simulink model "Plant_s"  (R2023a)
settings: Solver=VariableStepAuto  StartTime=0.0  StopTime=10.0  RelTol=1e-3
undefined symbols (not defined in the file): c, C, C_alpha_f, C_col, C_r, E, e_p0, F_zf, F_zr, Iz, J_col, K, l_f, l_r, m, n_st, T_f
settings Model: Creator=Tan_Tram  LastModifiedBy=Tan_Tram

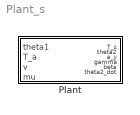
== system Plant_s ==
  Plant : Subsystem

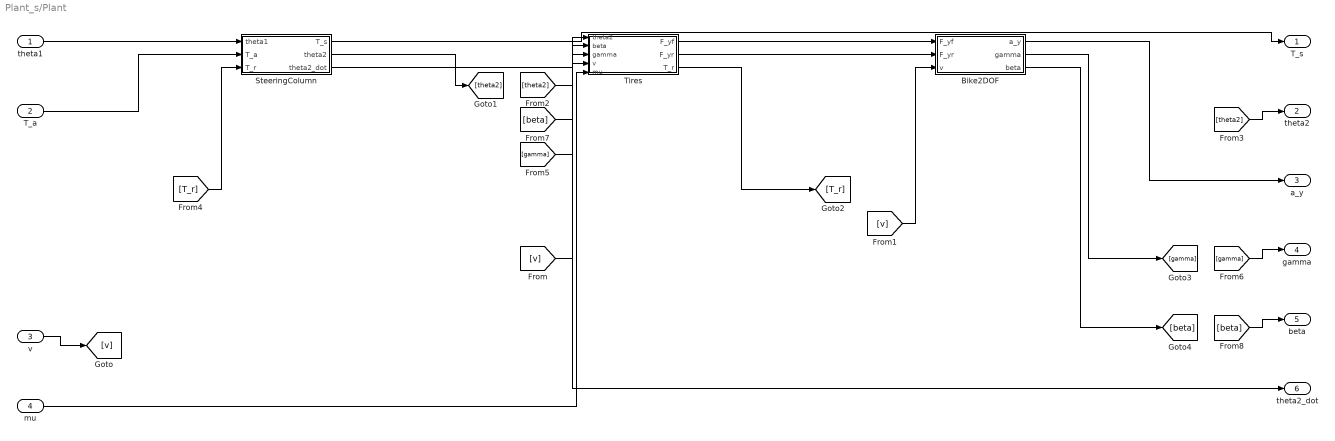
== system Plant_s/Plant ==
  theta1 : Inport
  T_a : Inport  Port=2
  v : Inport  Port=3
  mu : Inport  Port=4
  Bike2DOF : Subsystem
  SteeringColumn : Subsystem
  Tires : Subsystem
  T_s : Outport
  theta2 : Outport  Port=2
  a_y : Outport  Port=3
  gamma : Outport  Port=4
  beta : Outport  Port=5
  theta2_dot : Outport  Port=6
  wires:
  theta1/1 -> SteeringColumn/1(theta1)
  T_a/1 -> SteeringColumn/2(T_a)
  mu/1 -> Tires/5(mu)
  Tires/1(F_yf) -> Bike2DOF/1(F_yf)
  Tires/2(F_yr) -> Bike2DOF/2(F_yr)
  SteeringColumn/1(T_s) -> T_s/1
  Bike2DOF/1(a_y) -> a_y/1
  SteeringColumn/3(theta2_dot) -> theta2_dot/1
  v/1 -> [v]
  [v] -> Tires/4(v)
  [v] -> Bike2DOF/3(v)
  SteeringColumn/2(theta2) -> [theta2]
  [theta2] -> Tires/1(theta2)
  [theta2] -> theta2/1
  Tires/3(T_r) -> [T_r]
  [T_r] -> SteeringColumn/3(T_r)
  Bike2DOF/2(gamma) -> [gamma]
  [gamma] -> Tires/3(gamma)
  [gamma] -> gamma/1
  Bike2DOF/3(beta) -> [beta]
  [beta] -> Tires/2(beta)
  [beta] -> beta/1

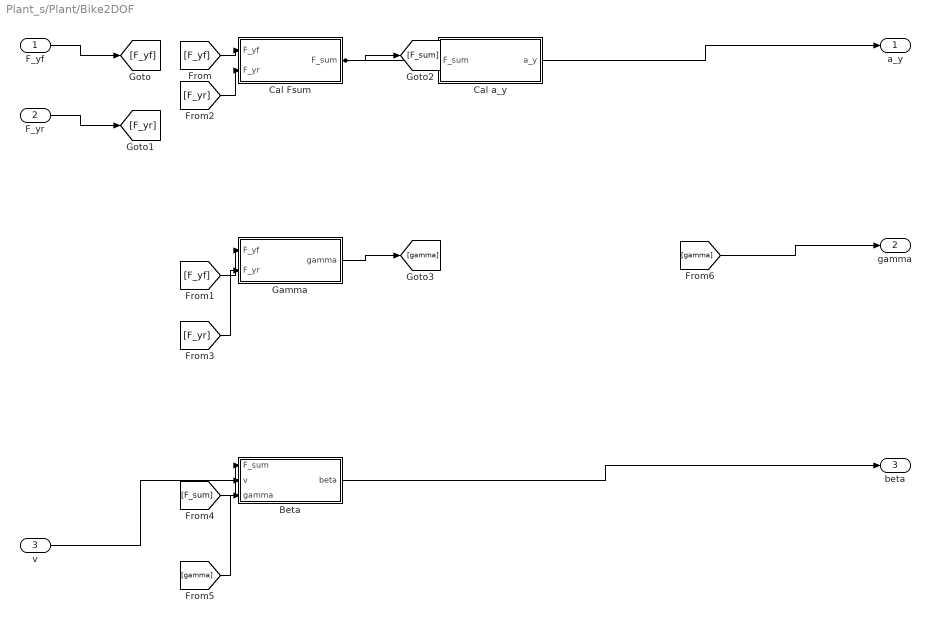
== system Plant_s/Plant/Bike2DOF ==
  F_yf : Inport
  F_yr : Inport  Port=2
  v : Inport  Port=3
  Beta : Subsystem
  Cal Fsum : Subsystem
  Cal a_y : Subsystem
  Gamma : Subsystem
  a_y : Outport
  gamma : Outport  Port=2
  beta : Outport  Port=3
  wires:
  Beta/1(beta) -> beta/1
  v/1 -> Beta/2(v)
  [gamma] -> gamma/1
  [gamma] -> Beta/3(gamma)
  Gamma/1(gamma) -> [gamma]
  Cal a_y/1(a_y) -> a_y/1
  [F_sum] -> Beta/1(F_sum)
  Cal Fsum/1(F_sum) -> [F_sum], Cal a_y/1(F_sum)
  [F_yr] -> Gamma/2(F_yr)
  [F_yr] -> Cal Fsum/2(F_yr)
  F_yr/1 -> [F_yr]
  [F_yf] -> Gamma/1(F_yf)
  [F_yf] -> Cal Fsum/1(F_yf)
  F_yf/1 -> [F_yf]

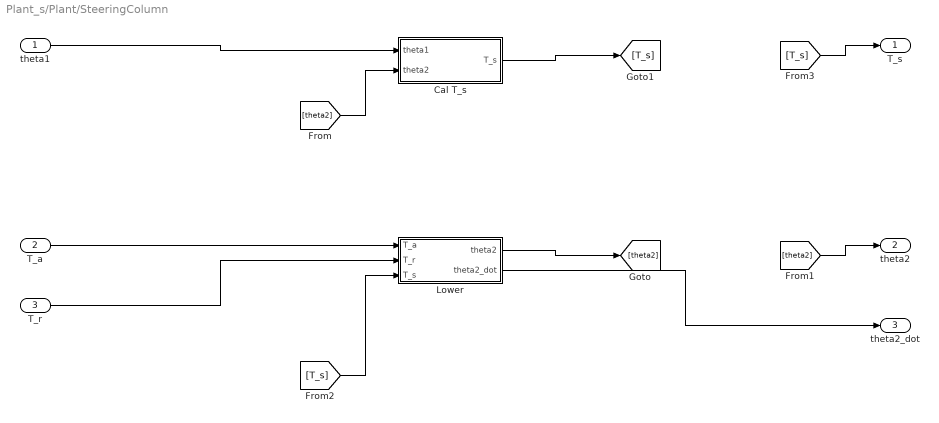
== system Plant_s/Plant/SteeringColumn ==
  theta1 : Inport
  T_a : Inport  Port=2
  T_r : Inport  Port=3
  Cal T_s : Subsystem
  Lower : Subsystem
  T_s : Outport
  theta2 : Outport  Port=2
  theta2_dot : Outport  Port=3
  wires:
  [T_s] -> T_s/1
  [T_s] -> Lower/3(T_s)
  Cal T_s/1(T_s) -> [T_s]
  [theta2] -> theta2/1
  [theta2] -> Cal T_s/2(theta2)
  Lower/1(theta2) -> [theta2]
  Lower/2(theta2_dot) -> theta2_dot/1
  T_r/1 -> Lower/2(T_r)
  T_a/1 -> Lower/1(T_a)
  theta1/1 -> Cal T_s/1(theta1)

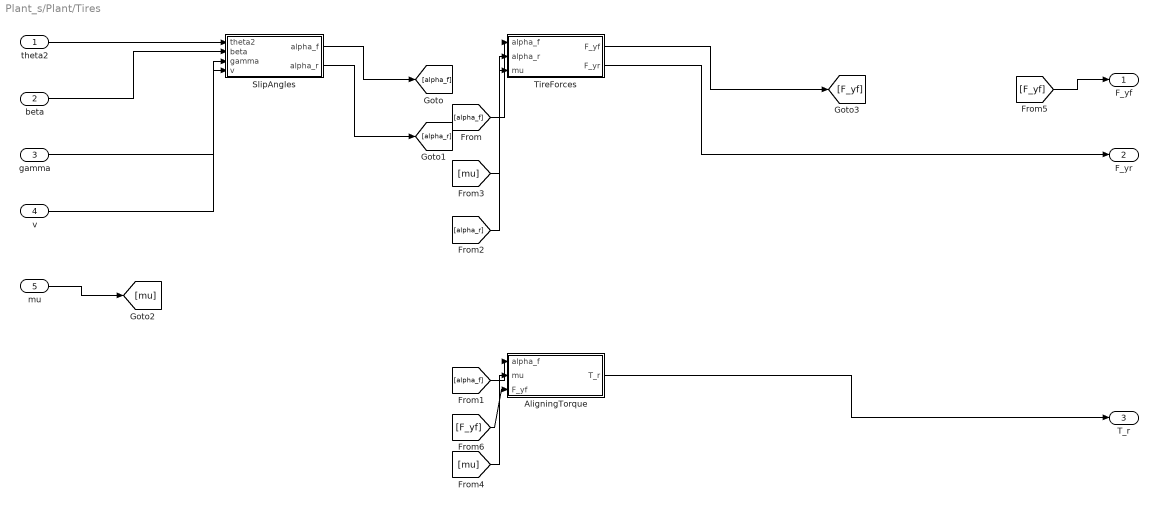
== system Plant_s/Plant/Tires ==
  theta2 : Inport
  beta : Inport  Port=2
  gamma : Inport  Port=3
  v : Inport  Port=4
  mu : Inport  Port=5
  AligningTorque : Subsystem
  SlipAngles : Subsystem
  TireForces : Subsystem
  F_yf : Outport
  F_yr : Outport  Port=2
  T_r : Outport  Port=3
  wires:
  AligningTorque/1(T_r) -> T_r/1
  TireForces/2(F_yr) -> F_yr/1
  [F_yf] -> AligningTorque/3(F_yf)
  [F_yf] -> F_yf/1
  TireForces/1(F_yf) -> [F_yf]
  [mu] -> AligningTorque/2(mu)
  [mu] -> TireForces/3(mu)
  mu/1 -> [mu]
  [alpha_r] -> TireForces/2(alpha_r)
  SlipAngles/2(alpha_r) -> [alpha_r]
  [alpha_f] -> AligningTorque/1(alpha_f)
  [alpha_f] -> TireForces/1(alpha_f)
  SlipAngles/1(alpha_f) -> [alpha_f]
  v/1 -> SlipAngles/4(v)
  gamma/1 -> SlipAngles/3(gamma)
  beta/1 -> SlipAngles/2(beta)
  theta2/1 -> SlipAngles/1(theta2)

== system Plant_s/Plant/Bike2DOF/Beta ==
  F_sum : Inport
  v : Inport  Port=2
  gamma : Inport  Port=3
  Constant : Constant  Value=m
  Div_Fsum_mv : Product  Inputs=*/
  Int_beta : Integrator
  Prod_mv : Product  Inputs=**
  Sum_betadot : Sum  Inputs=+-
  beta : Outport
  wires:
  Int_beta/1 -> beta/1
  Sum_betadot/1 -> Int_beta/1
  gamma/1 -> Sum_betadot/2
  Div_Fsum_mv/1 -> Sum_betadot/1
  Prod_mv/1 -> Div_Fsum_mv/2
  F_sum/1 -> Div_Fsum_mv/1
  v/1 -> Prod_mv/2
  Constant/1 -> Prod_mv/1

== system Plant_s/Plant/Bike2DOF/Cal Fsum ==
  F_yf : Inport
  F_yr : Inport  Port=2
  Sum_Fsum : Sum
  F_sum : Outport
  wires:
  Sum_Fsum/1 -> F_sum/1
  F_yr/1 -> Sum_Fsum/2
  F_yf/1 -> Sum_Fsum/1

== system Plant_s/Plant/Bike2DOF/Cal a_y ==
  F_sum : Inport
  Constant : Constant  Value=m
  Div_ay : Product  Inputs=*/
  a_y : Outport
  wires:
  Div_ay/1 -> a_y/1
  Constant/1 -> Div_ay/2
  F_sum/1 -> Div_ay/1

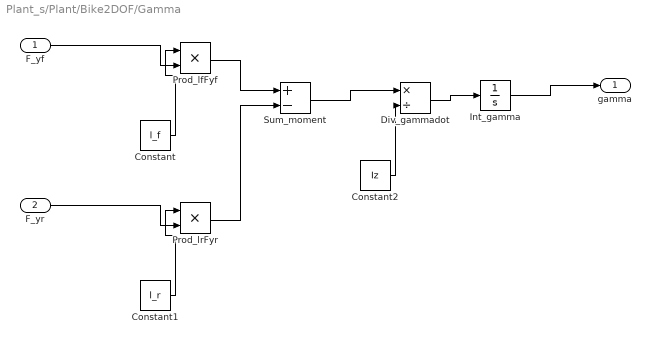
== system Plant_s/Plant/Bike2DOF/Gamma ==
  F_yf : Inport
  F_yr : Inport  Port=2
  Constant : Constant  Value=l_f
  Constant1 : Constant  Value=l_r
  Constant2 : Constant  Value=Iz
  Div_gammadot : Product  Inputs=*/
  Int_gamma : Integrator
  Prod_lfFyf : Product  Inputs=**
  Prod_lrFyr : Product  Inputs=**
  Sum_moment : Sum  Inputs=+-
  gamma : Outport
  wires:
  Int_gamma/1 -> gamma/1
  Div_gammadot/1 -> Int_gamma/1
  Constant2/1 -> Div_gammadot/2
  Sum_moment/1 -> Div_gammadot/1
  Prod_lrFyr/1 -> Sum_moment/2
  Prod_lfFyf/1 -> Sum_moment/1
  F_yr/1 -> Prod_lrFyr/2
  Constant1/1 -> Prod_lrFyr/1
  F_yf/1 -> Prod_lfFyf/2
  Constant/1 -> Prod_lfFyf/1

== system Plant_s/Plant/SteeringColumn/Cal T_s ==
  theta1 : Inport
  theta2 : Inport  Port=2
  Constant : Constant  Value=K
  Prod_Ts : Product  Inputs=**
  Sum_dTheta : Sum  Inputs=+-
  T_s : Outport
  wires:
  Prod_Ts/1 -> T_s/1
  Constant/1 -> Prod_Ts/2
  Sum_dTheta/1 -> Prod_Ts/1
  theta2/1 -> Sum_dTheta/2
  theta1/1 -> Sum_dTheta/1

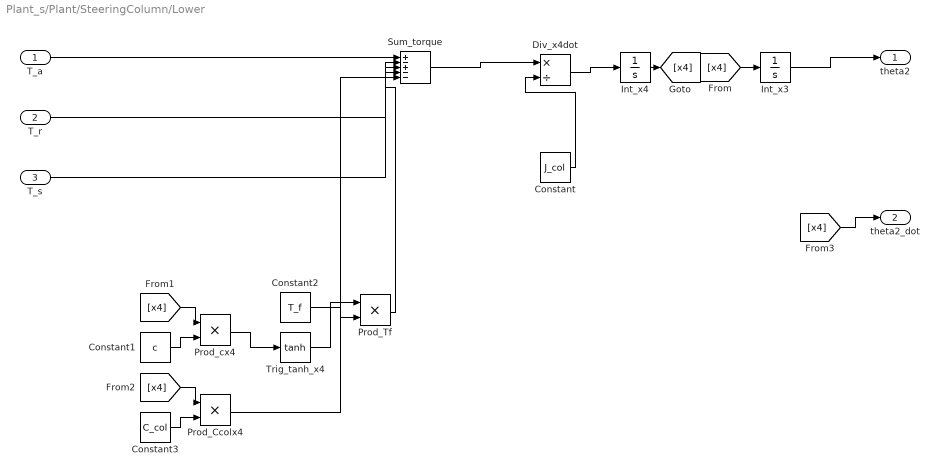
== system Plant_s/Plant/SteeringColumn/Lower ==
  T_a : Inport
  T_r : Inport  Port=2
  T_s : Inport  Port=3
  Constant : Constant  Value=J_col
  Constant1 : Constant  Value=c
  Constant2 : Constant  Value=T_f
  Constant3 : Constant  Value=C_col
  Div_x4dot : Product  Inputs=*/
  Int_x3 : Integrator
  Int_x4 : Integrator
  Prod_Ccolx4 : Product  Inputs=**
  Prod_Tf : Product  Inputs=**
  Prod_cx4 : Product  Inputs=**
  Sum_torque : Sum  Inputs=+-+--
  Trig_tanh_x4 : Trigonometry  Operator=tanh
  theta2 : Outport
  theta2_dot : Outport  Port=2
  wires:
  [x4] -> theta2_dot/1
  Int_x3/1 -> theta2/1
  [x4] -> Int_x3/1
  Div_x4dot/1 -> Int_x4/1
  Constant/1 -> Div_x4dot/2
  Sum_torque/1 -> Div_x4dot/1
  Prod_Ccolx4/1 -> Sum_torque/5
  Prod_Tf/1 -> Sum_torque/4
  T_s/1 -> Sum_torque/3
  T_r/1 -> Sum_torque/2
  T_a/1 -> Sum_torque/1
  Constant3/1 -> Prod_Ccolx4/2
  [x4] -> Prod_Ccolx4/1
  Constant2/1 -> Prod_Tf/2
  Trig_tanh_x4/1 -> Prod_Tf/1
  Prod_cx4/1 -> Trig_tanh_x4/1
  Constant1/1 -> Prod_cx4/2
  [x4] -> Prod_cx4/1
  Int_x4/1 -> [x4]

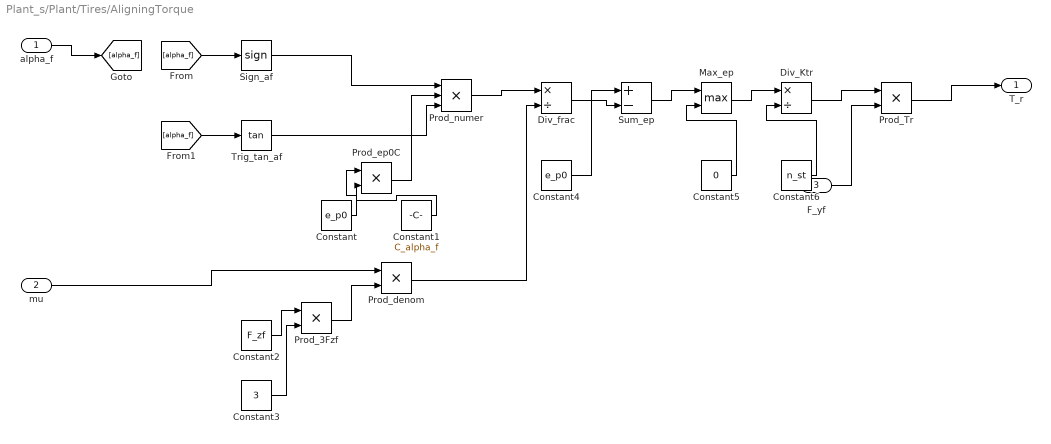
== system Plant_s/Plant/Tires/AligningTorque ==
  alpha_f : Inport
  mu : Inport  Port=2
  F_yf : Inport  Port=3
  Constant : Constant  Value=e_p0
  Constant1 : Constant  Value=C_alpha_f
  Constant2 : Constant  Value=F_zf
  Constant3 : Constant  Value=3
  Constant4 : Constant  Value=e_p0
  Constant5 : Constant  Value=0
  Constant6 : Constant  Value=n_st
  Div_Ktr : Product  Inputs=*/
  Div_frac : Product  Inputs=*/
  Max_ep : MinMax  Function=max  Inputs=2
  Prod_3Fzf : Product  Inputs=**
  Prod_Tr : Product  Inputs=**
  Prod_denom : Product  Inputs=**
  Prod_ep0C : Product  Inputs=**
  Prod_numer : Product  Inputs=***
  Sign_af : Signum
  Sum_ep : Sum  Inputs=+-
  Trig_tan_af : Trigonometry  Operator=tan
  T_r : Outport
  wires:
  Prod_Tr/1 -> T_r/1
  F_yf/1 -> Prod_Tr/2
  Div_Ktr/1 -> Prod_Tr/1
  Constant6/1 -> Div_Ktr/2
  Max_ep/1 -> Div_Ktr/1
  Constant5/1 -> Max_ep/2
  Sum_ep/1 -> Max_ep/1
  Div_frac/1 -> Sum_ep/2
  Constant4/1 -> Sum_ep/1
  Prod_denom/1 -> Div_frac/2
  Prod_numer/1 -> Div_frac/1
  Prod_3Fzf/1 -> Prod_denom/2
  mu/1 -> Prod_denom/1
  Constant3/1 -> Prod_3Fzf/2
  Constant2/1 -> Prod_3Fzf/1
  Trig_tan_af/1 -> Prod_numer/3
  Prod_ep0C/1 -> Prod_numer/2
  Sign_af/1 -> Prod_numer/1
  Constant1/1 -> Prod_ep0C/2
  Constant/1 -> Prod_ep0C/1
  [alpha_f] -> Trig_tan_af/1
  [alpha_f] -> Sign_af/1
  alpha_f/1 -> [alpha_f]

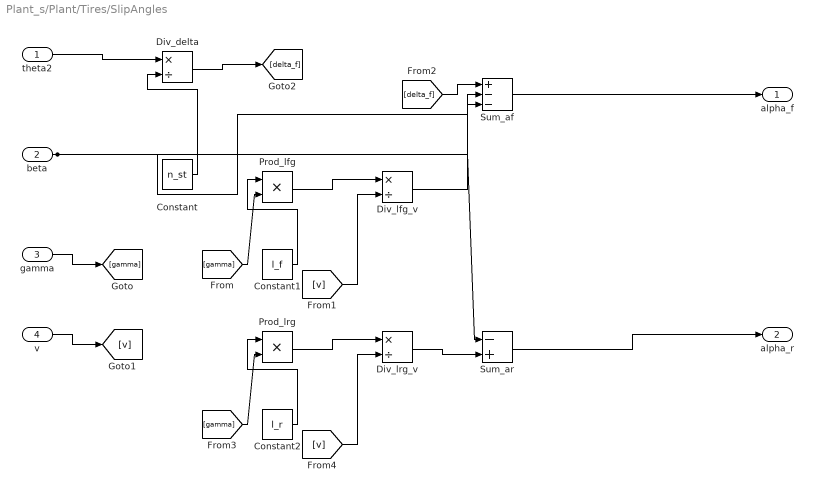
== system Plant_s/Plant/Tires/SlipAngles ==
  theta2 : Inport
  beta : Inport  Port=2
  gamma : Inport  Port=3
  v : Inport  Port=4
  Constant : Constant  Value=n_st
  Constant1 : Constant  Value=l_f
  Constant2 : Constant  Value=l_r
  Div_delta : Product  Inputs=*/
  Div_lfg_v : Product  Inputs=*/
  Div_lrg_v : Product  Inputs=*/
  Prod_lfg : Product  Inputs=**
  Prod_lrg : Product  Inputs=**
  Sum_af : Sum  Inputs=+--
  Sum_ar : Sum  Inputs=-+
  alpha_f : Outport
  alpha_r : Outport  Port=2
  wires:
  Sum_ar/1 -> alpha_r/1
  Div_lrg_v/1 -> Sum_ar/2
  [v] -> Div_lrg_v/2
  Prod_lrg/1 -> Div_lrg_v/1
  [gamma] -> Prod_lrg/2
  Constant2/1 -> Prod_lrg/1
  Sum_af/1 -> alpha_f/1
  Div_lfg_v/1 -> Sum_af/3
  beta/1 -> Sum_ar/1, Sum_af/2
  [delta_f] -> Sum_af/1
  Div_delta/1 -> [delta_f]
  [v] -> Div_lfg_v/2
  Prod_lfg/1 -> Div_lfg_v/1
  [gamma] -> Prod_lfg/2
  Constant1/1 -> Prod_lfg/1
  Constant/1 -> Div_delta/2
  theta2/1 -> Div_delta/1
  v/1 -> [v]
  gamma/1 -> [gamma]

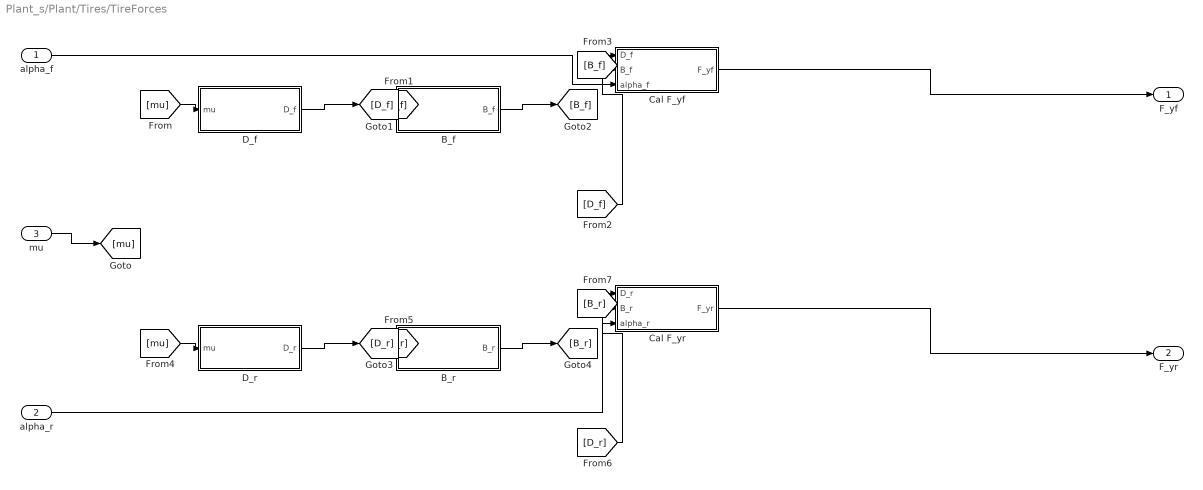
== system Plant_s/Plant/Tires/TireForces ==
  alpha_f : Inport
  alpha_r : Inport  Port=2
  mu : Inport  Port=3
  B_f : Subsystem
  B_r : Subsystem
  Cal F_yf : Subsystem
  Cal F_yr : Subsystem
  D_f : Subsystem
  D_r : Subsystem
  F_yf : Outport
  F_yr : Outport  Port=2
  wires:
  Cal F_yr/1(F_yr) -> F_yr/1
  alpha_r/1 -> Cal F_yr/3(alpha_r)
  [B_r] -> Cal F_yr/2(B_r)
  B_r/1(B_r) -> [B_r]
  [D_r] -> Cal F_yr/1(D_r)
  [D_r] -> B_r/1(D_r)
  D_r/1(D_r) -> [D_r]
  [mu] -> D_r/1(mu)
  Cal F_yf/1(F_yf) -> F_yf/1
  alpha_f/1 -> Cal F_yf/3(alpha_f)
  [B_f] -> Cal F_yf/2(B_f)
  B_f/1(B_f) -> [B_f]
  [D_f] -> Cal F_yf/1(D_f)
  [D_f] -> B_f/1(D_f)
  D_f/1(D_f) -> [D_f]
  [mu] -> D_f/1(mu)
  mu/1 -> [mu]

== system Plant_s/Plant/Tires/TireForces/B_f ==
  D_f : Inport
  Constant : Constant  Value=C
  Constant1 : Constant  Value=C_alpha_f
  Div_B : Product  Inputs=*/
  Prod_CD : Product  Inputs=**
  B_f : Outport
  wires:
  Div_B/1 -> B_f/1
  Prod_CD/1 -> Div_B/2
  Constant1/1 -> Div_B/1
  Constant/1 -> Prod_CD/2
  D_f/1 -> Prod_CD/1

== system Plant_s/Plant/Tires/TireForces/B_r ==
  D_r : Inport
  Constant : Constant  Value=C
  Constant1 : Constant  Value=C_r
  Div_B : Product  Inputs=*/
  Prod_CD : Product  Inputs=**
  B_r : Outport
  wires:
  Div_B/1 -> B_r/1
  Prod_CD/1 -> Div_B/2
  Constant1/1 -> Div_B/1
  Constant/1 -> Prod_CD/2
  D_r/1 -> Prod_CD/1

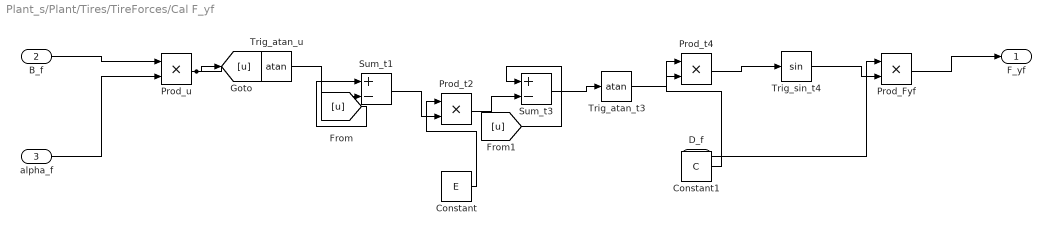
== system Plant_s/Plant/Tires/TireForces/Cal F_yf ==
  D_f : Inport
  B_f : Inport  Port=2
  alpha_f : Inport  Port=3
  Constant : Constant  Value=E
  Constant1 : Constant  Value=C
  Prod_Fyf : Product  Inputs=**
  Prod_t2 : Product  Inputs=**
  Prod_t4 : Product  Inputs=**
  Prod_u : Product  Inputs=**
  Sum_t1 : Sum  Inputs=+-
  Sum_t3 : Sum  Inputs=+-
  Trig_atan_t3 : Trigonometry  Operator=atan
  Trig_atan_u : Trigonometry  Operator=atan
  Trig_sin_t4 : Trigonometry
  F_yf : Outport
  wires:
  Prod_Fyf/1 -> F_yf/1
  Trig_sin_t4/1 -> Prod_Fyf/2
  D_f/1 -> Prod_Fyf/1
  Prod_t4/1 -> Trig_sin_t4/1
  Trig_atan_t3/1 -> Prod_t4/2
  Constant1/1 -> Prod_t4/1
  Sum_t3/1 -> Trig_atan_t3/1
  Prod_t2/1 -> Sum_t3/2
  [u] -> Sum_t3/1
  Sum_t1/1 -> Prod_t2/2
  Constant/1 -> Prod_t2/1
  Trig_atan_u/1 -> Sum_t1/2
  [u] -> Sum_t1/1
  Prod_u/1 -> [u], Trig_atan_u/1
  alpha_f/1 -> Prod_u/2
  B_f/1 -> Prod_u/1

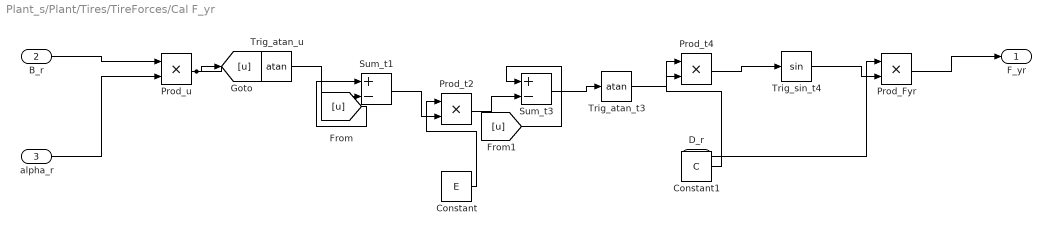
== system Plant_s/Plant/Tires/TireForces/Cal F_yr ==
  D_r : Inport
  B_r : Inport  Port=2
  alpha_r : Inport  Port=3
  Constant : Constant  Value=E
  Constant1 : Constant  Value=C
  Prod_Fyr : Product  Inputs=**
  Prod_t2 : Product  Inputs=**
  Prod_t4 : Product  Inputs=**
  Prod_u : Product  Inputs=**
  Sum_t1 : Sum  Inputs=+-
  Sum_t3 : Sum  Inputs=+-
  Trig_atan_t3 : Trigonometry  Operator=atan
  Trig_atan_u : Trigonometry  Operator=atan
  Trig_sin_t4 : Trigonometry
  F_yr : Outport
  wires:
  Prod_Fyr/1 -> F_yr/1
  Trig_sin_t4/1 -> Prod_Fyr/2
  D_r/1 -> Prod_Fyr/1
  Prod_t4/1 -> Trig_sin_t4/1
  Trig_atan_t3/1 -> Prod_t4/2
  Constant1/1 -> Prod_t4/1
  Sum_t3/1 -> Trig_atan_t3/1
  Prod_t2/1 -> Sum_t3/2
  [u] -> Sum_t3/1
  Sum_t1/1 -> Prod_t2/2
  Constant/1 -> Prod_t2/1
  Trig_atan_u/1 -> Sum_t1/2
  [u] -> Sum_t1/1
  Prod_u/1 -> [u], Trig_atan_u/1
  alpha_r/1 -> Prod_u/2
  B_r/1 -> Prod_u/1

== system Plant_s/Plant/Tires/TireForces/D_f ==
  mu : Inport
  Constant : Constant  Value=F_zf
  Prod_D : Product  Inputs=**
  D_f : Outport
  wires:
  Prod_D/1 -> D_f/1
  Constant/1 -> Prod_D/2
  mu/1 -> Prod_D/1

== system Plant_s/Plant/Tires/TireForces/D_r ==
  mu : Inport
  Constant : Constant  Value=F_zr
  Prod_D : Product  Inputs=**
  D_r : Outport
  wires:
  Prod_D/1 -> D_r/1
  Constant/1 -> Prod_D/2
  mu/1 -> Prod_D/1
